simulink model "DroneModelV2"  (R2023b)
settings: Solver=VariableStepAuto  StartTime=0.0  StopTime=time_model  RelTol=1e-3
values from neighbouring files (symbols this model uses):
  A_flap = [c_a, c_b, 0 ... (first row only)    [testModel.m]
  A_ind = [c_d, 0, 0 ... (first row only)    [testModel.m]
  C_drag = C_drag_arr(i)    [testModel.m]
  g = 9.8    [testModel.m]
  Ix = m/3*a^2/12+2*0.045*l^2    (= 0.00211347222222)    [testModel.m]
  Iy = m/3*a^2/12+4*0.045*l^2    (= 0.00413847222222)    [testModel.m]
  Iz = m/3*a^2/4+2*0.045*l^2    (= 0.00229041666667)    [testModel.m]
  J = 2.5*10^(-6)    (= 2.5e-06)    [testModel.m]
  Ke = ke    (= 0.0073)    [testModel.m]
  kf = ks*r^2*airDensity*Sblade/2    (= 1.57565625e-05)    [testModel.m]
  Km = kt    (= 0.0073)    [testModel.m]
  L = La    (= 5e-05)    [testModel.m]
  l = 0.15    [testModel.m]
  m = 0.65    [testModel.m]
  maxU = 11    [testModel.m]
  R = ra    (= 0.048)    [testModel.m]
  rho = 1.225    [testModel.m]
  S = l*c*4+a*b    (= 0.0169)    [testModel.m]
  U1 = U1_arr(i)    [testModel.m]
  U2 = U2_arr(i)    [testModel.m]
  U3 = U3_arr(i)    [testModel.m]
  U4 = U4_arr(i)    [testModel.m]
libraries: sharedtransform x1
settings Model: Creator=Degra  LastModifiedBy=Degra

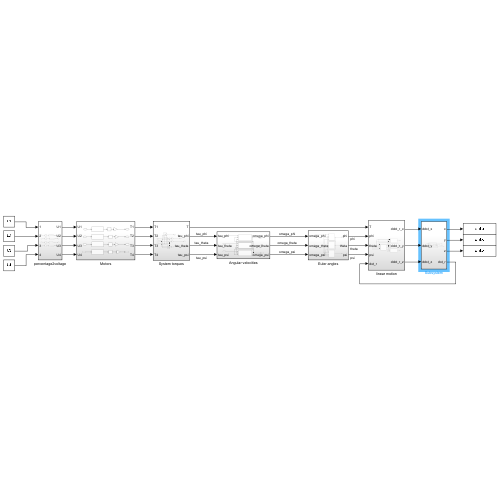
[thumbnail: Simulink's stored preview of the top-level diagram]
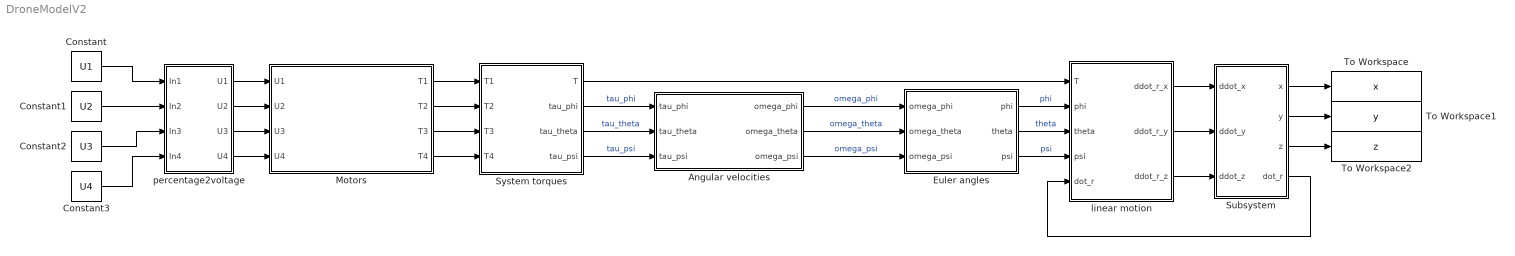
== system DroneModelV2 ==
  Angular velocities : Subsystem
  Constant : Constant  Value=U1
  Constant1 : Constant  Value=U2
  Constant2 : Constant  Value=U3
  Constant3 : Constant  Value=U4
  Euler angles : Subsystem
  Motors : Subsystem
  Subsystem : Subsystem
  System torques : Subsystem
  To Workspace : ToWorkspace  VariableName=x  SaveFormat=Timeseries  SampleTime=-1
  To Workspace1 : ToWorkspace  VariableName=y  SaveFormat=Timeseries  SampleTime=-1
  To Workspace2 : ToWorkspace  VariableName=z  SaveFormat=Timeseries  SampleTime=-1
  linear motion : Subsystem
  percentage2voltage : Subsystem
  wires:
  Motors/1(T1) -> System torques/1(T1)
  Motors/2(T2) -> System torques/2(T2)
  Motors/3(T3) -> System torques/3(T3)
  Motors/4(T4) -> System torques/4(T4)
  System torques/2(tau_phi) -> Angular velocities/1(tau_phi)  "tau_phi"
  System torques/3(tau_theta) -> Angular velocities/2(tau_theta)  "tau_theta"
  System torques/4(tau_psi) -> Angular velocities/3(tau_psi)  "tau_psi"
  Angular velocities/1(omega_phi) -> Euler angles/1(omega_phi)  "omega_phi"
  Angular velocities/2(omega_theta) -> Euler angles/2(omega_theta)  "omega_theta"
  Angular velocities/3(omega_psi) -> Euler angles/3(omega_psi)  "omega_psi"
  Euler angles/1(phi) -> linear motion/2(phi)  "phi"
  Euler angles/2(theta) -> linear motion/3(theta)  "theta"
  Euler angles/3(psi) -> linear motion/4(psi)  "psi"
  System torques/1(T) -> linear motion/1(T)
  Constant/1 -> percentage2voltage/1(In1)
  Constant1/1 -> percentage2voltage/2(In2)
  Constant2/1 -> percentage2voltage/3(In3)
  Constant3/1 -> percentage2voltage/4(In4)
  percentage2voltage/1(U1) -> Motors/1(U1)
  percentage2voltage/2(U2) -> Motors/2(U2)
  percentage2voltage/3(U3) -> Motors/3(U3)
  percentage2voltage/4(U4) -> Motors/4(U4)
  linear motion/1(ddot_r_x) -> Subsystem/1(ddot_x)
  linear motion/2(ddot_r_y) -> Subsystem/2(ddot_y)
  linear motion/3(ddot_r_z) -> Subsystem/3(ddot_z)
  Subsystem/1(x) -> To Workspace/1
  Subsystem/2(y) -> To Workspace1/1
  Subsystem/4(dot_r) -> linear motion/5(dot_r)
  Subsystem/3(z) -> To Workspace2/1

== system DroneModelV2/Angular velocities ==
  tau_phi : Inport
  tau_theta : Inport  Port=2
  tau_psi : Inport  Port=3
  Subsystem1 : Subsystem
  Subsystem2 : Subsystem
  Subsystem3 : Subsystem
  omega_phi : Outport
  omega_theta : Outport  Port=2
  omega_psi : Outport  Port=3
  wires:
  Subsystem2/1(omega_theta) -> omega_theta/1, Subsystem1/2(omega_theta), Subsystem3/3(omega_theta)  "omega_theta"
  tau_theta/1 -> Subsystem2/1(tau_theta)
  Subsystem1/1(omega_phi) -> omega_phi/1, Subsystem3/2(omega_phi), Subsystem2/2(omega_phi)  "omega_phi"
  Subsystem3/1(omega_psi) -> omega_psi/1, Subsystem2/3(omega_psi), Subsystem1/3(omega_psi)  "omega_psi"
  tau_phi/1 -> Subsystem1/1(tau_phi)
  tau_psi/1 -> Subsystem3/1(tau_psi)

== system DroneModelV2/Euler angles ==
  omega_phi : Inport
  omega_theta : Inport  Port=2
  omega_psi : Inport  Port=3
  Subsystem1 : Subsystem
  Subsystem2 : Subsystem
  Subsystem3 : Subsystem
  phi : Outport
  theta : Outport  Port=2
  psi : Outport  Port=3
  wires:
  Subsystem2/1(theta) -> theta/1, Subsystem1/2(theta), Subsystem3/4(theta)  "theta"
  Subsystem1/1(phi) -> phi/1, Subsystem3/1(phi), Subsystem2/1(phi)  "phi"
  omega_theta/1 -> Subsystem3/2(omega_theta), Subsystem1/3(omega_theta), Subsystem2/2(omega_theta)
  omega_psi/1 -> Subsystem2/3(omega_psi), Subsystem3/3(omega_psi), Subsystem1/4(omega_psi)
  omega_phi/1 -> Subsystem1/1(omega_phi)
  Subsystem3/1(psi) -> psi/1  "psi"

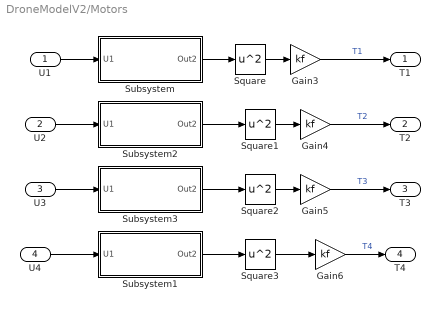
== system DroneModelV2/Motors ==
  U1 : Inport
  U2 : Inport  Port=2
  U3 : Inport  Port=3
  U4 : Inport  Port=4
  Gain{3..6} (4 alike) : Gain  Gain=kf
  Square{,1..3} (4 alike) : Math  Operator=square
  Subsystem : Subsystem
  Subsystem1 : Subsystem
  Subsystem2 : Subsystem
  Subsystem3 : Subsystem
  T1 : Outport
  T2 : Outport  Port=2
  T3 : Outport  Port=3
  T4 : Outport  Port=4
  wires:
  Square2/1 -> Gain5/1
  Square/1 -> Gain3/1
  Square1/1 -> Gain4/1
  Square3/1 -> Gain6/1
  Subsystem3/1(Out2) -> Square2/1
  U4/1 -> Subsystem1/1(U1)
  U1/1 -> Subsystem/1(U1)
  Gain6/1 -> T4/1  "T4"
  U3/1 -> Subsystem3/1(U1)
  Gain3/1 -> T1/1  "T1"
  Gain4/1 -> T2/1  "T2"
  Gain5/1 -> T3/1  "T3"
  Subsystem1/1(Out2) -> Square3/1
  U2/1 -> Subsystem2/1(U1)
  Subsystem2/1(Out2) -> Square1/1
  Subsystem/1(Out2) -> Square/1

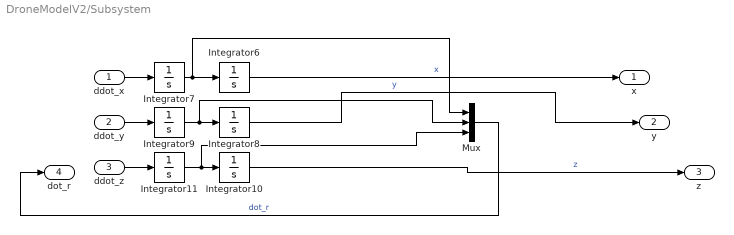
== system DroneModelV2/Subsystem ==
  ddot_x : Inport
  ddot_y : Inport  Port=2
  ddot_z : Inport  Port=3
  Integrator10 : Integrator  InitialCondition=100
  Integrator11 : Integrator
  Integrator6 : Integrator  InitialCondition=100
  Integrator7 : Integrator
  Integrator8 : Integrator  InitialCondition=100
  Integrator9 : Integrator
  Mux : Mux  Inputs=3
  x : Outport
  y : Outport  Port=2
  z : Outport  Port=3
  dot_r : Outport  Port=4
  wires:
  Integrator9/1 -> Mux/2, Integrator8/1
  Integrator7/1 -> Mux/1, Integrator6/1
  Integrator10/1 -> z/1  "z"
  Integrator11/1 -> Mux/3, Integrator10/1
  Integrator8/1 -> y/1  "y"
  ddot_x/1 -> Integrator7/1
  Mux/1 -> dot_r/1  "dot_r"
  Integrator6/1 -> x/1  "x"
  ddot_y/1 -> Integrator9/1
  ddot_z/1 -> Integrator11/1

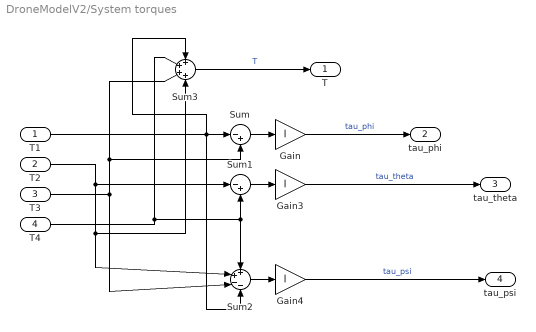
== system DroneModelV2/System torques ==
  T1 : Inport
  T2 : Inport  Port=2
  T3 : Inport  Port=3
  T4 : Inport  Port=4
  Gain : Gain  Gain=l
  Gain3 : Gain  Gain=l
  Gain4 : Gain  Gain=l
  Sum : Sum  Inputs=|-+
  Sum1 : Sum  Inputs=|-+
  Sum2 : Sum  Inputs=++--
  Sum3 : Sum  Inputs=++++
  T : Outport
  tau_phi : Outport  Port=2
  tau_theta : Outport  Port=3
  tau_psi : Outport  Port=4
  wires:
  T3/1 -> Sum2/3, Sum3/3, Sum/2
  T4/1 -> Sum3/2, Sum1/2, Sum2/1
  Sum2/1 -> Gain4/1
  Gain4/1 -> tau_psi/1  "tau_psi"
  T1/1 -> Sum2/4, Sum3/1, Sum/1
  Sum/1 -> Gain/1
  Sum1/1 -> Gain3/1
  Sum3/1 -> T/1  "T"
  T2/1 -> Sum2/2, Sum3/4, Sum1/1
  Gain3/1 -> tau_theta/1  "tau_theta"
  Gain/1 -> tau_phi/1  "tau_phi"

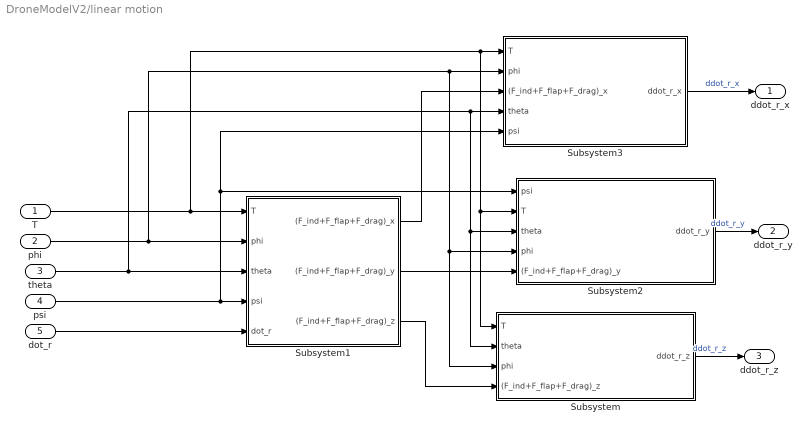
== system DroneModelV2/linear motion ==
  T : Inport
  phi : Inport  Port=2
  theta : Inport  Port=3
  psi : Inport  Port=4
  dot_r : Inport  Port=5
  Subsystem : Subsystem
  Subsystem1 : Subsystem
  Subsystem2 : Subsystem
  Subsystem3 : Subsystem
  ddot_r_x : Outport
  ddot_r_y : Outport  Port=2
  ddot_r_z : Outport  Port=3
  wires:
  T/1 -> Subsystem/1(T), Subsystem2/2(T), Subsystem3/1(T), Subsystem1/1(T)
  theta/1 -> Subsystem/2(theta), Subsystem2/3(theta), Subsystem3/4(theta), Subsystem1/3(theta)
  phi/1 -> Subsystem/3(phi), Subsystem2/4(phi), Subsystem3/2(phi), Subsystem1/2(phi)
  Subsystem1/3((F_ind+F_flap+F_drag)_z) -> Subsystem/4((F_ind+F_flap+F_drag)_z)
  psi/1 -> Subsystem3/5(psi), Subsystem2/1(psi), Subsystem1/4(psi)
  dot_r/1 -> Subsystem1/5(dot_r)
  Subsystem1/2((F_ind+F_flap+F_drag)_y) -> Subsystem2/5((F_ind+F_flap+F_drag)_y)
  Subsystem1/1((F_ind+F_flap+F_drag)_x) -> Subsystem3/3((F_ind+F_flap+F_drag)_x)
  Subsystem3/1(ddot_r_x) -> ddot_r_x/1  "ddot_r_x"
  Subsystem2/1(ddot_r_y) -> ddot_r_y/1  "ddot_r_y"
  Subsystem/1(ddot_r_z) -> ddot_r_z/1  "ddot_r_z"

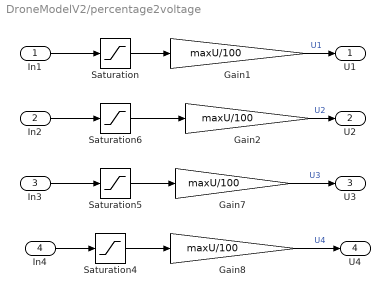
== system DroneModelV2/percentage2voltage ==
  In1 : Inport
  In2 : Inport  Port=2
  In3 : Inport  Port=3
  In4 : Inport  Port=4
  Gain{1..2,7..8} (4 alike) : Gain  Gain=maxU/100
  Saturation{,4..6} (4 alike) : Saturate  UpperLimit=100  LowerLimit=-100
  U1 : Outport
  U2 : Outport  Port=2
  U3 : Outport  Port=3
  U4 : Outport  Port=4
  wires:
  In4/1 -> Saturation4/1
  Gain7/1 -> U3/1  "U3"
  Saturation5/1 -> Gain7/1
  In1/1 -> Saturation/1
  Saturation4/1 -> Gain8/1
  Saturation6/1 -> Gain2/1
  Gain1/1 -> U1/1  "U1"
  Saturation/1 -> Gain1/1
  Gain2/1 -> U2/1  "U2"
  Gain8/1 -> U4/1  "U4"
  In2/1 -> Saturation6/1
  In3/1 -> Saturation5/1

== system DroneModelV2/Angular velocities/Subsystem1 ==
  tau_phi : Inport
  omega_theta : Inport  Port=2
  omega_psi : Inport  Port=3
  Gain : Gain  Gain=Iz-Iy
  Integrator12 : Integrator
  Product : Product
  Sum : Sum  Inputs=|++
  omega_phi : Outport
  wires:
  Gain/1 -> Sum/2
  Integrator12/1 -> omega_phi/1  "omega_phi"
  omega_theta/1 -> Product/1
  Product/1 -> Gain/1
  Sum/1 -> Integrator12/1  "dot_omega_phi"
  tau_phi/1 -> Sum/1
  omega_psi/1 -> Product/2

== system DroneModelV2/Angular velocities/Subsystem2 ==
  tau_theta : Inport
  omega_phi : Inport  Port=2
  omega_psi : Inport  Port=3
  Gain : Gain  Gain=Ix-Iz
  Integrator12 : Integrator
  Product : Product
  Sum : Sum  Inputs=|++
  omega_theta : Outport
  wires:
  Gain/1 -> Sum/2
  Integrator12/1 -> omega_theta/1  "omega_theta"
  omega_phi/1 -> Product/1
  Product/1 -> Gain/1
  Sum/1 -> Integrator12/1  "dot_omega_theta"
  tau_theta/1 -> Sum/1
  omega_psi/1 -> Product/2

== system DroneModelV2/Angular velocities/Subsystem3 ==
  tau_psi : Inport
  omega_phi : Inport  Port=2
  omega_theta : Inport  Port=3
  Gain : Gain  Gain=Iy-Ix
  Integrator12 : Integrator
  Product : Product
  Sum : Sum  Inputs=|++
  omega_psi : Outport
  wires:
  Gain/1 -> Sum/2
  Integrator12/1 -> omega_psi/1  "omega_psi"
  omega_phi/1 -> Product/1
  Product/1 -> Gain/1
  Sum/1 -> Integrator12/1  "dot_omega_psi"
  tau_psi/1 -> Sum/1
  omega_theta/1 -> Product/2

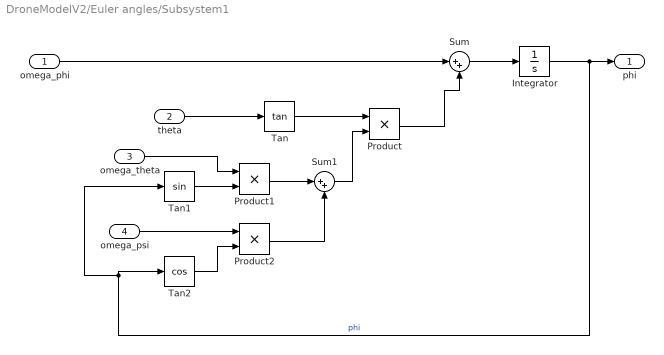
== system DroneModelV2/Euler angles/Subsystem1 ==
  omega_phi : Inport
  theta : Inport  Port=2
  omega_theta : Inport  Port=3
  omega_psi : Inport  Port=4
  Integrator : Integrator
  Product : Product
  Product1 : Product
  Product2 : Product
  Sum : Sum  Inputs=|++
  Sum1 : Sum  Inputs=|++
  Tan : Trigonometry  Operator=tan
  Tan1 : Trigonometry
  Tan2 : Trigonometry  Operator=cos
  phi : Outport
  wires:
  Product2/1 -> Sum1/2
  Tan1/1 -> Product1/2
  Sum/1 -> Integrator/1
  Sum1/1 -> Product/2
  Tan/1 -> Product/1
  Tan2/1 -> Product2/2
  Product1/1 -> Sum1/1
  Product/1 -> Sum/2
  omega_psi/1 -> Product2/1
  omega_theta/1 -> Product1/1
  Integrator/1 -> Tan1/1, Tan2/1, phi/1  "phi"
  theta/1 -> Tan/1
  omega_phi/1 -> Sum/1

== system DroneModelV2/Euler angles/Subsystem2 ==
  phi : Inport
  omega_theta : Inport  Port=2
  omega_psi : Inport  Port=3
  Integrator : Integrator
  Product1 : Product
  Product2 : Product
  Sum1 : Sum  Inputs=|+-
  Tan1 : Trigonometry  Operator=cos
  Tan2 : Trigonometry
  theta : Outport
  wires:
  Product2/1 -> Sum1/2
  Tan1/1 -> Product1/2
  Tan2/1 -> Product2/2
  Product1/1 -> Sum1/1
  Sum1/1 -> Integrator/1
  omega_psi/1 -> Product2/1
  omega_theta/1 -> Product1/1
  Integrator/1 -> theta/1  "theta"
  phi/1 -> Tan2/1, Tan1/1

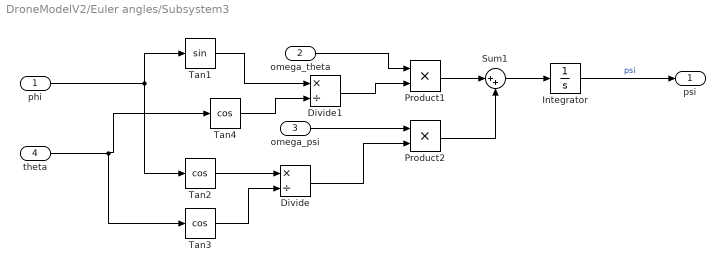
== system DroneModelV2/Euler angles/Subsystem3 ==
  phi : Inport
  omega_theta : Inport  Port=2
  omega_psi : Inport  Port=3
  theta : Inport  Port=4
  Divide : Product  Inputs=*/
  Divide1 : Product  Inputs=*/
  Integrator : Integrator
  Product1 : Product
  Product2 : Product
  Sum1 : Sum  Inputs=|++
  Tan1 : Trigonometry
  Tan2 : Trigonometry  Operator=cos
  Tan3 : Trigonometry  Operator=cos
  Tan4 : Trigonometry  Operator=cos
  psi : Outport
  wires:
  Product2/1 -> Sum1/2
  Product1/1 -> Sum1/1
  Sum1/1 -> Integrator/1
  omega_psi/1 -> Product2/1
  omega_theta/1 -> Product1/1
  Integrator/1 -> psi/1  "psi"
  phi/1 -> Tan1/1, Tan2/1
  theta/1 -> Tan4/1, Tan3/1
  Divide/1 -> Product2/2
  Tan2/1 -> Divide/1
  Tan3/1 -> Divide/2
  Divide1/1 -> Product1/2
  Tan1/1 -> Divide1/1
  Tan4/1 -> Divide1/2

== system DroneModelV2/Motors/Subsystem ==
  U1 : Inport
  Add : Sum  Inputs=+--
  Gain2 : Gain  Gain=1/L
  Gain3 : Gain  Gain=Ke
  Gain4 : Gain  Gain=Km/J
  Gain5 : Gain  Gain=R
  Integrator : Integrator
  Integrator2 : Integrator
  Out2 : Outport
  wires:
  Gain2/1 -> Integrator/1
  Gain3/1 -> Add/2
  Add/1 -> Gain2/1
  Gain4/1 -> Integrator2/1
  Integrator/1 -> Gain4/1, Gain5/1
  Gain5/1 -> Add/3
  U1/1 -> Add/1
  Integrator2/1 -> Out2/1, Gain3/1

== system DroneModelV2/Motors/Subsystem1 ==
  U1 : Inport
  Add : Sum  Inputs=+--
  Gain1 : Gain  Gain=1/J
  Gain2 : Gain  Gain=1/L
  Gain3 : Gain  Gain=Ke
  Gain4 : Gain  Gain=Km
  Gain5 : Gain  Gain=R
  Integrator : Integrator
  Integrator2 : Integrator
  Sum : Sum  Inputs=|+-
  Out2 : Outport
  wires:
  Gain2/1 -> Integrator/1
  Gain3/1 -> Add/2
  Add/1 -> Gain2/1
  Integrator/1 -> Gain4/1, Gain5/1
  Gain5/1 -> Add/3
  U1/1 -> Add/1
  Integrator2/1 -> Out2/1, Gain3/1
  Gain1/1 -> Integrator2/1
  Gain4/1 -> Sum/1
  Sum/1 -> Gain1/1
  ? -> Sum/2

== system DroneModelV2/Motors/Subsystem2 ==
  U1 : Inport
  Add : Sum  Inputs=+--
  Gain2 : Gain  Gain=1/L
  Gain3 : Gain  Gain=Ke
  Gain4 : Gain  Gain=Km/J
  Gain5 : Gain  Gain=R
  Integrator : Integrator
  Integrator2 : Integrator
  Out2 : Outport
  wires:
  Gain2/1 -> Integrator/1
  Gain3/1 -> Add/2
  Add/1 -> Gain2/1
  Gain4/1 -> Integrator2/1
  Integrator/1 -> Gain4/1, Gain5/1
  Gain5/1 -> Add/3
  U1/1 -> Add/1
  Integrator2/1 -> Out2/1, Gain3/1

== system DroneModelV2/Motors/Subsystem3 ==
  U1 : Inport
  Add : Sum  Inputs=+--
  Gain2 : Gain  Gain=1/L
  Gain3 : Gain  Gain=Ke
  Gain4 : Gain  Gain=Km/J
  Gain5 : Gain  Gain=R
  Integrator : Integrator
  Integrator2 : Integrator
  Out2 : Outport
  wires:
  Gain2/1 -> Integrator/1
  Gain3/1 -> Add/2
  Add/1 -> Gain2/1
  Gain4/1 -> Integrator2/1
  Integrator/1 -> Gain4/1, Gain5/1
  Gain5/1 -> Add/3
  U1/1 -> Add/1
  Integrator2/1 -> Out2/1, Gain3/1

== system DroneModelV2/linear motion/Subsystem ==
  T : Inport
  theta : Inport  Port=2
  phi : Inport  Port=3
  (F_ind+F_flap+F_drag)_z : Inport  Port=4
  Constant4 : Constant  Value=m*g
  Cos4 : Trigonometry  Operator=cos
  Cos5 : Trigonometry  Operator=cos
  Gain4 : Gain  Gain=1/m
  Product2 : Product  Inputs=3
  Sum2 : Sum  Inputs=|+--
  ddot_r_z : Outport
  wires:
  Product2/1 -> Sum2/1
  phi/1 -> Cos4/1
  theta/1 -> Cos5/1
  T/1 -> Product2/1
  Cos4/1 -> Product2/2
  Constant4/1 -> Sum2/3
  Cos5/1 -> Product2/3
  (F_ind+F_flap+F_drag)_z/1 -> Sum2/2
  Sum2/1 -> Gain4/1
  Gain4/1 -> ddot_r_z/1  "ddot_r_z"

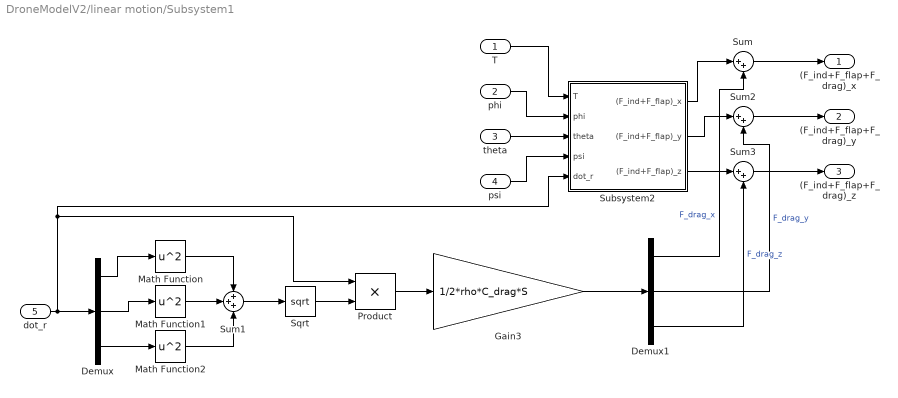
== system DroneModelV2/linear motion/Subsystem1 ==
  T : Inport
  phi : Inport  Port=2
  theta : Inport  Port=3
  psi : Inport  Port=4
  dot_r : Inport  Port=5
  Demux : Demux  Outputs=3
  Demux1 : Demux  Outputs=3
  Gain3 : Gain  Gain=1/2*rho*C_drag*S
  Math Function : Math  Operator=square
  Math Function1 : Math  Operator=square
  Math Function2 : Math  Operator=square
  Product : Product
  Sqrt : Sqrt
  Subsystem2 : Subsystem
  Sum : Sum  Inputs=|++
  Sum1 : Sum  Inputs=+++
  Sum2 : Sum  Inputs=|++
  Sum3 : Sum  Inputs=|++
  (F_ind+F_flap+F_drag)_x : Outport
  (F_ind+F_flap+F_drag)_y : Outport  Port=2
  (F_ind+F_flap+F_drag)_z : Outport  Port=3
  wires:
  Demux1/2 -> Sum2/2  "F_drag_y"
  dot_r/1 -> Product/1, Subsystem2/5(dot_r), Demux/1
  Math Function1/1 -> Sum1/2
  Demux/1 -> Math Function/1
  Demux/2 -> Math Function1/1
  Sum1/1 -> Sqrt/1
  Math Function/1 -> Sum1/1
  Demux/3 -> Math Function2/1
  Demux1/3 -> Sum3/2  "F_drag_z"
  Subsystem2/2((F_ind+F_flap)_y) -> Sum2/1
  Math Function2/1 -> Sum1/3
  Sqrt/1 -> Product/2
  phi/1 -> Subsystem2/2(phi)
  Product/1 -> Gain3/1
  T/1 -> Subsystem2/1(T)
  theta/1 -> Subsystem2/3(theta)
  psi/1 -> Subsystem2/4(psi)
  Gain3/1 -> Demux1/1
  Subsystem2/1((F_ind+F_flap)_x) -> Sum/1
  Subsystem2/3((F_ind+F_flap)_z) -> Sum3/1
  Demux1/1 -> Sum/2  "F_drag_x"
  Sum/1 -> (F_ind+F_flap+F_drag)_x/1
  Sum2/1 -> (F_ind+F_flap+F_drag)_y/1
  Sum3/1 -> (F_ind+F_flap+F_drag)_z/1

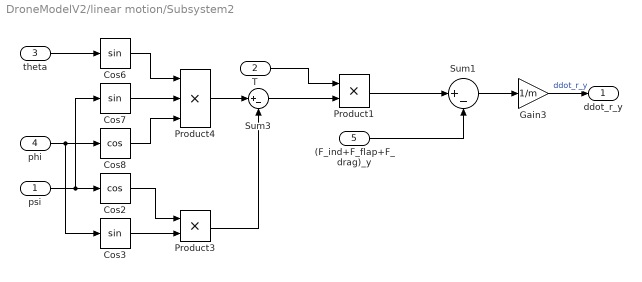
== system DroneModelV2/linear motion/Subsystem2 ==
  psi : Inport
  T : Inport  Port=2
  theta : Inport  Port=3
  phi : Inport  Port=4
  (F_ind+F_flap+F_drag)_y : Inport  Port=5
  Cos2 : Trigonometry  Operator=cos
  Cos3 : Trigonometry
  Cos6 : Trigonometry
  Cos7 : Trigonometry
  Cos8 : Trigonometry  Operator=cos
  Gain3 : Gain  Gain=1/m
  Product1 : Product
  Product3 : Product
  Product4 : Product  Inputs=3
  Sum1 : Sum  Inputs=|+-
  Sum3 : Sum  Inputs=|+-
  ddot_r_y : Outport
  wires:
  Cos6/1 -> Product4/1
  theta/1 -> Cos6/1
  psi/1 -> Cos7/1, Cos2/1
  Cos7/1 -> Product4/2
  Sum1/1 -> Gain3/1
  phi/1 -> Cos3/1, Cos8/1
  Cos8/1 -> Product4/3
  Cos2/1 -> Product3/1
  Cos3/1 -> Product3/2
  Product4/1 -> Sum3/1
  Product3/1 -> Sum3/2
  T/1 -> Product1/1
  Sum3/1 -> Product1/2
  Product1/1 -> Sum1/1
  (F_ind+F_flap+F_drag)_y/1 -> Sum1/2
  Gain3/1 -> ddot_r_y/1  "ddot_r_y"

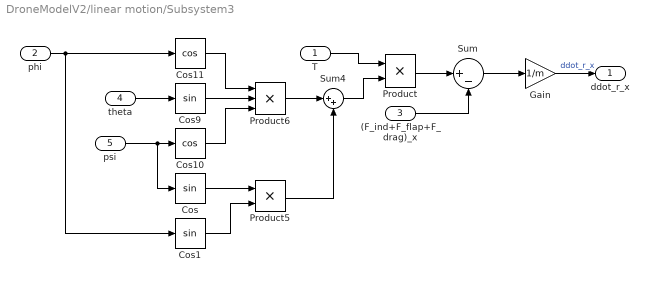
== system DroneModelV2/linear motion/Subsystem3 ==
  T : Inport
  phi : Inport  Port=2
  (F_ind+F_flap+F_drag)_x : Inport  Port=3
  theta : Inport  Port=4
  psi : Inport  Port=5
  Cos : Trigonometry
  Cos1 : Trigonometry
  Cos10 : Trigonometry  Operator=cos
  Cos11 : Trigonometry  Operator=cos
  Cos9 : Trigonometry
  Gain : Gain  Gain=1/m
  Product : Product
  Product5 : Product
  Product6 : Product  Inputs=3
  Sum : Sum  Inputs=|+-
  Sum4 : Sum  Inputs=|++
  ddot_r_x : Outport
  wires:
  theta/1 -> Cos9/1
  Cos/1 -> Product5/1
  psi/1 -> Cos10/1, Cos/1
  Cos11/1 -> Product6/1
  Sum/1 -> Gain/1
  (F_ind+F_flap+F_drag)_x/1 -> Sum/2
  phi/1 -> Cos11/1, Cos1/1
  Cos1/1 -> Product5/2
  Cos9/1 -> Product6/2
  Cos10/1 -> Product6/3
  Product6/1 -> Sum4/1
  Product5/1 -> Sum4/2
  T/1 -> Product/1
  Sum4/1 -> Product/2
  Product/1 -> Sum/1
  Gain/1 -> ddot_r_x/1  "ddot_r_x"

== system DroneModelV2/linear motion/Subsystem1/Subsystem2 ==
  T : Inport
  phi : Inport  Port=2
  theta : Inport  Port=3
  psi : Inport  Port=4
  dot_r : Inport  Port=5
  Demux : Demux  Outputs=3
  Subsystem1 : Subsystem
  (F_ind+F_flap)_x : Outport
  (F_ind+F_flap)_y : Outport  Port=2
  (F_ind+F_flap)_z : Outport  Port=3
  wires:
  T/1 -> Subsystem1/5(T)
  Subsystem1/1(F_ind+F_flap) -> Demux/1
  psi/1 -> Subsystem1/3(psi)
  Demux/2 -> (F_ind+F_flap)_y/1  "(F_ind+F_flap)_y"
  dot_r/1 -> Subsystem1/4(dot_r)
  theta/1 -> Subsystem1/2(theta)
  phi/1 -> Subsystem1/1(phi)
  Demux/1 -> (F_ind+F_flap)_x/1  "(F_ind+F_flap)_x"
  Demux/3 -> (F_ind+F_flap)_z/1  "(F_ind+F_flap)_z"

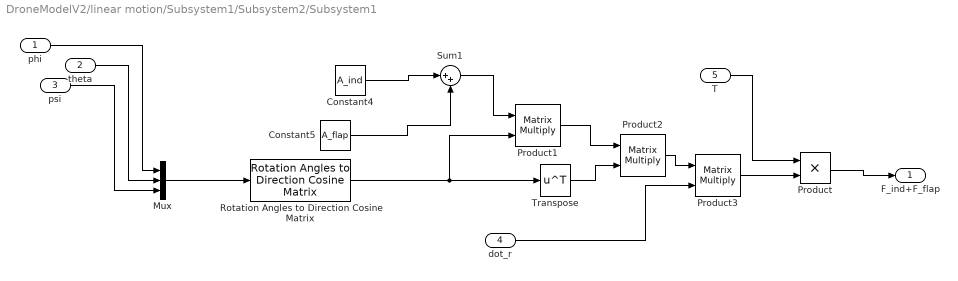
== system DroneModelV2/linear motion/Subsystem1/Subsystem2/Subsystem1 ==
  phi : Inport
  theta : Inport  Port=2
  psi : Inport  Port=3
  dot_r : Inport  Port=4
  T : Inport  Port=5
  Constant4 : Constant  Value=A_ind
  Constant5 : Constant  Value=A_flap
  Mux : Mux  Inputs=3
  Product : Product
  Product1 : Product  Multiplication=Matrix(*)
  Product2 : Product  Multiplication=Matrix(*)
  Product3 : Product  Multiplication=Matrix(*)
  Rotation Angles to Direction Cosine Matrix : sharedtransform/Rotation Angles to Direction Cosine Matrix  rotationOrder=ZYX  aMode=aMode
  Sum1 : Sum  Inputs=|++
  Transpose : Math  Operator=transpose
  F_ind+F_flap : Outport
  wires:
  Constant4/1 -> Sum1/1
  Product1/1 -> Product2/1
  Sum1/1 -> Product1/1
  Constant5/1 -> Sum1/2
  psi/1 -> Mux/3
  Product2/1 -> Product3/1
  Rotation Angles to Direction Cosine Matrix/1 -> Product1/2, Transpose/1
  theta/1 -> Mux/2
  Mux/1 -> Rotation Angles to Direction Cosine Matrix/1
  Transpose/1 -> Product2/2
  phi/1 -> Mux/1
  dot_r/1 -> Product3/2
  Product3/1 -> Product/2
  Product/1 -> F_ind+F_flap/1
  T/1 -> Product/1
